simulink model "BASK"  (R2021a)
settings: Solver=VariableStepAuto  StartTime=0.0  StopTime=0.005  RelTol=1e-3
libraries: dsparch4 x2, commchan3 x1, commrandsrc3 x1, commsink2 x1
settings Model: Creator=MrCai  LastModifiedBy=MrCai

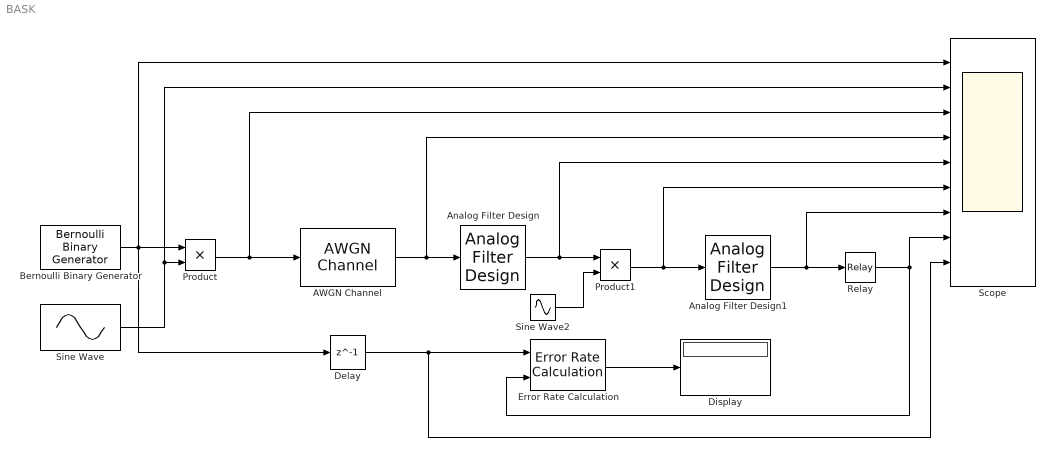
== system BASK ==
  AWGN Channel : commchan3/AWGN Channel  InputProcessing=Columns as channels (frame based)  seed=67  noiseMode="Signal to noise ratio  (SNR)"  EbNodB=10  EsNodB=10  SNRdB=2  bitsPerSym=1  Ps=1  Tsym=1  variance=1
  Analog Filter Design : dsparch4/Analog Filter Design  method=Butterworth  filttype=Bandpass  N=8  Wlo=2*pi*90*1000  Whi=2*pi*110*1000  Rp=2  Rs=40
  Analog Filter Design1 : dsparch4/Analog Filter Design  method=Butterworth  filttype=Lowpass  N=8  Wlo=2*pi*110*1000  Whi=80  Rp=2  Rs=40
  Bernoulli Binary Generator : commrandsrc3/Bernoulli Binary Generator  ProbabilityOfZero=0.5  SeedSource=Auto  Seed=0  SampleTime=1/10000  SamplesPerFrame=1  OutputDataType=double  SimulateUsing=Interpreted execution
  Delay : Delay  DelayLength=1
  Display : Display
  Error Rate Calculation : commsink2/Error Rate Calculation  N=0  st_delay=0  cp_mode=Entire frame  subframe=[]  PMode=Port  WsName=ErrorVec  RsMode2=off  stop=off  numErr=100  maxBits=1e6
  Product : Product
  Product1 : Product
  Relay : Relay  OnSwitchValue=0.25  OffSwitchValue=0.25
  Scope : Scope  NumInputPorts=9
  Sine Wave : Sin  Frequency=2*pi*100*1000  SampleTime=1/1000000
  Sine Wave2 : Sin  Frequency=2*pi*100*1000  SampleTime=1/1000000
  wires:
  Bernoulli Binary Generator/1 -> Scope/1, Delay/1, Product/1
  Sine Wave/1 -> Scope/2, Product/2
  Product/1 -> AWGN Channel/1, Scope/3
  Analog Filter Design/1 -> Scope/5, Product1/1
  Product1/1 -> Scope/6, Analog Filter Design1/1
  Analog Filter Design1/1 -> Scope/7, Relay/1
  Sine Wave2/1 -> Product1/2
  Relay/1 -> Error Rate Calculation/2, Scope/8
  Error Rate Calculation/1 -> Display/1
  AWGN Channel/1 -> Scope/4, Analog Filter Design/1
  Delay/1 -> Scope/9, Error Rate Calculation/1
